simulink model "inverted_pendulum_deadbeat"  (R2020a)
settings: Solver=VariableStepAuto  StartTime=0.0  StopTime=0.4  MaxStep=1e-1  RelTol=1e-3
undefined symbols (not defined in the file): C, c, g, gam, h, Jt, Kdeadbeat, L, m, Mt
settings Model: Creator=TomJa  LastModifiedBy=TomJa

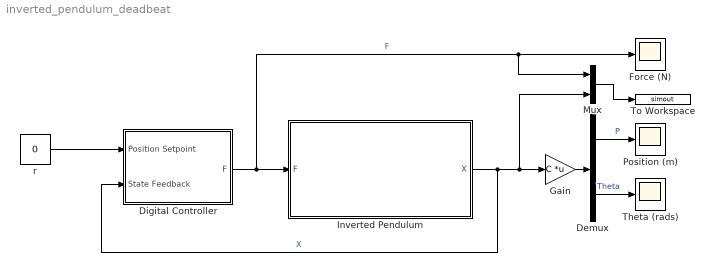
== system inverted_pendulum_deadbeat ==
  Demux : Demux  Outputs=2
  Digital Controller : Subsystem
  Force (N) : Scope
  Gain : Gain  Gain=C  Multiplication=Matrix(K*u)
  Inverted Pendulum : Subsystem
  Mux : Mux  Inputs=2
  Position (m) : Scope
  Theta (rads) : Scope
  To Workspace : ToWorkspace  VariableName=simout  SaveFormat=Timeseries  SampleTime=-1
  r : Constant  Value=0
  wires:
  Digital Controller/1(F) -> Mux/1, Force (N)/1, Inverted Pendulum/1(F)  "F"
  r/1 -> Digital Controller/1(Position Setpoint)
  Inverted Pendulum/1(X) -> Mux/2, Gain/1, Digital Controller/2(State Feedback)  "X"
  Demux/1 -> Position (m)/1  "P"
  Demux/2 -> Theta (rads)/1  "Theta"
  Gain/1 -> Demux/1
  Mux/1 -> To Workspace/1

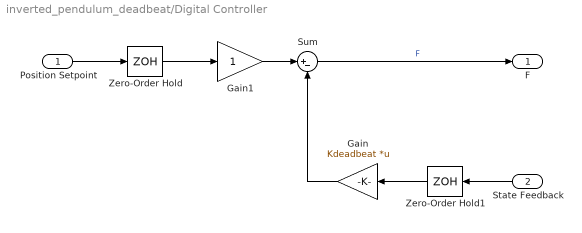
== system inverted_pendulum_deadbeat/Digital Controller ==
  Position Setpoint : Inport
  State Feedback : Inport  Port=2
  Gain : Gain  Gain=Kdeadbeat  Multiplication=Matrix(K*u)
  Gain1 : Gain
  Sum : Sum  Inputs=|+-
  Zero-Order Hold : ZeroOrderHold  SampleTime=h
  Zero-Order Hold1 : ZeroOrderHold  SampleTime=h
  F : Outport  PortDimensions=1
  wires:
  Gain1/1 -> Sum/1
  State Feedback/1 -> Zero-Order Hold1/1
  Position Setpoint/1 -> Zero-Order Hold/1
  Zero-Order Hold/1 -> Gain1/1
  Zero-Order Hold1/1 -> Gain/1
  Gain/1 -> Sum/2
  Sum/1 -> F/1  "F"

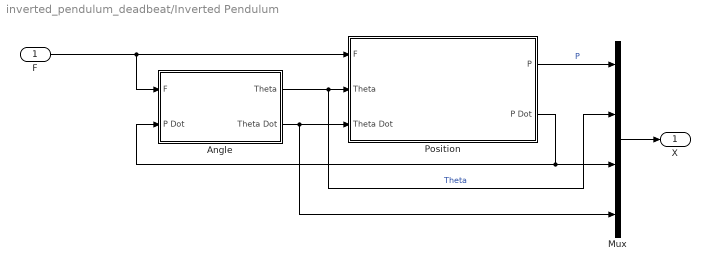
== system inverted_pendulum_deadbeat/Inverted Pendulum ==
  F : Inport
  Angle : Subsystem
  Mux : Mux
  Position : Subsystem
  X : Outport
  wires:
  Angle/1(Theta) -> Mux/2, Position/2(Theta)  "Theta"
  Position/2(P Dot) -> Angle/2(P Dot), Mux/3
  Angle/2(Theta Dot) -> Mux/4, Position/3(Theta Dot)
  Position/1(P) -> Mux/1  "P"
  F/1 -> Position/1(F), Angle/1(F)
  Mux/1 -> X/1

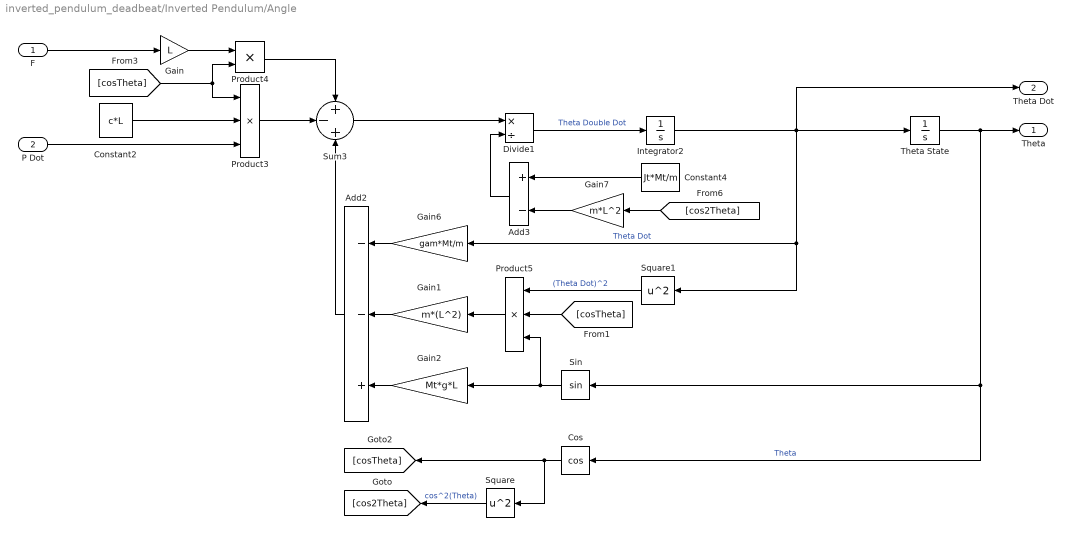
== system inverted_pendulum_deadbeat/Inverted Pendulum/Angle ==
  F : Inport  PortDimensions=1
  P Dot : Inport  Port=2  PortDimensions=1
  Add2 : Sum  Inputs=--+
  Add3 : Sum  Inputs=+-
  Constant2 : Constant  Value=c*L
  Constant4 : Constant  Value=Jt*Mt/m
  Cos : Trigonometry  Operator=cos
  Divide1 : Product  Inputs=*/
  Gain : Gain  Gain=L
  Gain1 : Gain  Gain=m*(L^2)
  Gain2 : Gain  Gain=Mt*g*L
  Gain6 : Gain  Gain=gam*Mt/m
  Gain7 : Gain  Gain=m*L^2
  Integrator2 : Integrator
  Product3 : Product  Inputs=3
  Product4 : Product
  Product5 : Product  Inputs=3
  Sin : Trigonometry
  Square : Math  Operator=square  SaturateOnIntegerOverflow=on
  Square1 : Math  Operator=square  SaturateOnIntegerOverflow=on
  Sum3 : Sum  Inputs=+-+
  Theta State : Integrator  InitialCondition=0.2  WrapState=on
  Theta : Outport  PortDimensions=1
  Theta Dot : Outport  Port=2  PortDimensions=1
  wires:
  Cos/1 -> [cosTheta], Square/1
  Product5/1 -> Gain1/1
  Product4/1 -> Sum3/1
  Add3/1 -> Divide1/2
  Sin/1 -> Gain2/1, Product5/3
  Theta State/1 -> Theta/1, Cos/1, Sin/1  "Theta"
  Square/1 -> [cos2Theta]  "cos^2(Theta)"
  P Dot/1 -> Product3/3
  Integrator2/1 -> Gain6/1, Square1/1, Theta Dot/1, Theta State/1  "Theta Dot"
  Gain6/1 -> Add2/1
  [cos2Theta] -> Gain7/1
  Constant2/1 -> Product3/2
  Gain/1 -> Product4/1
  [cosTheta] -> Product5/2
  Add2/1 -> Sum3/3
  Square1/1 -> Product5/1  "(Theta Dot)^2"
  F/1 -> Gain/1
  Product3/1 -> Sum3/2
  [cosTheta] -> Product4/2, Product3/1
  Sum3/1 -> Divide1/1
  Gain7/1 -> Add3/2
  Divide1/1 -> Integrator2/1  "Theta Double Dot"
  Gain2/1 -> Add2/3
  Constant4/1 -> Add3/1
  Gain1/1 -> Add2/2

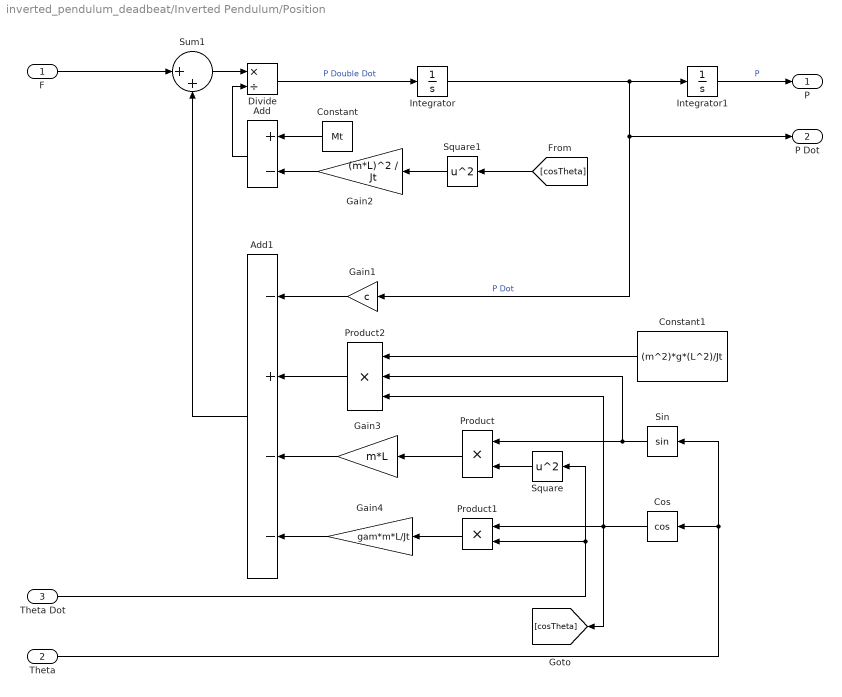
== system inverted_pendulum_deadbeat/Inverted Pendulum/Position ==
  F : Inport
  Theta : Inport  Port=2
  Theta Dot : Inport  Port=3
  Add : Sum  Inputs=+-
  Add1 : Sum  Inputs=-+--
  Constant : Constant  Value=Mt
  Constant1 : Constant  Value=(m^2)*g*(L^2)/Jt
  Cos : Trigonometry  Operator=cos
  Divide : Product  Inputs=*/
  Gain1 : Gain  Gain=c
  Gain2 : Gain  Gain=(m*L)^2 / Jt
  Gain3 : Gain  Gain=m*L
  Gain4 : Gain  Gain=gam*m*L/Jt
  Integrator : Integrator
  Integrator1 : Integrator  InitialCondition=0.1
  Product : Product
  Product1 : Product
  Product2 : Product  Inputs=3
  Sin : Trigonometry
  Square : Math  Operator=square  SaturateOnIntegerOverflow=on
  Square1 : Math  Operator=square  SaturateOnIntegerOverflow=on
  Sum1 : Sum  Inputs=|++
  P : Outport  PortDimensions=1
  P Dot : Outport  Port=2  PortDimensions=1
  wires:
  Constant/1 -> Add/1
  Sin/1 -> Product2/2, Product/1
  Product/1 -> Gain3/1
  Sum1/1 -> Divide/1
  Cos/1 -> [cosTheta], Product2/3, Product1/1
  Theta Dot/1 -> Square/1, Product1/2
  Gain1/1 -> Add1/1
  Add/1 -> Divide/2
  Gain2/1 -> Add/2
  Add1/1 -> Sum1/2
  Integrator/1 -> P Dot/1, Gain1/1, Integrator1/1  "P Dot"
  Gain3/1 -> Add1/3
  Gain4/1 -> Add1/4
  F/1 -> Sum1/1
  Product1/1 -> Gain4/1
  Product2/1 -> Add1/2
  Constant1/1 -> Product2/1
  Square/1 -> Product/2
  Integrator1/1 -> P/1  "P"
  Theta/1 -> Sin/1, Cos/1
  Square1/1 -> Gain2/1
  [cosTheta] -> Square1/1
  Divide/1 -> Integrator/1  "P Double Dot"
